simulink model "StateSpaceExeAntiWindup"  (Simulink 7.8)
settings: Solver=ode45  SolverMode=SingleTasking  StartTime=0.0  StopTime=50  RelTol=1e-3
values from neighbouring files (symbols this model uses):
  A = [-7.6258  0; 1  0]    [stateSpaceData.mat]
  B = [1 0]    [stateSpaceData.mat]
  C = [0 162.7435]    [stateSpaceData.mat]
  D = 0    [stateSpaceData.mat]
  K = [-1.6258 11]    [stateSpaceData.mat]    (also in toStateSpace.m = [Kx(1) Kx(2)]; toStateSpaceAntiWindup.m = [Kx(1) Kx(2)])
  Ki = 0.036867831895    [stateSpaceData.mat]    (also in toStateSpace.m = -Kx(3); toStateSpaceAntiWindup.m = -Kx(3))
  L = [80.8124614847 1.48930187688]    [stateSpaceData.mat]    (also in toStateSpace.m = acker(A', C', [polo1, polo2])'; toStateSpaceAntiWindup.m = acker(A', C', [polo1, polo2])')
settings Model: Creator=lucas  LastModifiedBy=lucas  CovMetricSettings=dwe  CovHtmlReporting=off  covSaveCumulativeToWorkspaceVar=off  CovSaveSingleToWorkspaceVar=off  CovExternalEMLEnable=on
settings DataIOCC: LimitDataPoints=off  SaveFormat=StructureWithTime  SignalLoggingSaveFormat=Dataset
settings OptimizationCC: ExpressionDepthLimit=128
settings DebuggingCC: UnderspecifiedInitializationDetection=Simplified  MergeDetectMultiDrivingBlocksExec=error  SolverPrmCheckMsg=none  FrameProcessingCompatibilityMsg=error  StateNameClashWarn=none  SFUnexpectedBacktrackingDiag=error  SFNoUnconditionalDefaultTransitionDiag=error
settings HardwareCC: ProdBitPerPointer=64  ProdLargestAtomicFloat=Float  ProdIntDivRoundTo=Zero  ProdEndianess=LittleEndian  ProdHWDeviceType=Specified
settings SFSimCC: SimUseLocalCustomCode=on
settings RTWCC: RTWUseLocalCustomCode=on
settings CodeAppCC: CustomSymbolStrType=$N$R$M_T
settings GRTTargetCC: TargetFunctionLibrary=C99 (ISO)  GeneratePreprocessorConditionals=Use local settings

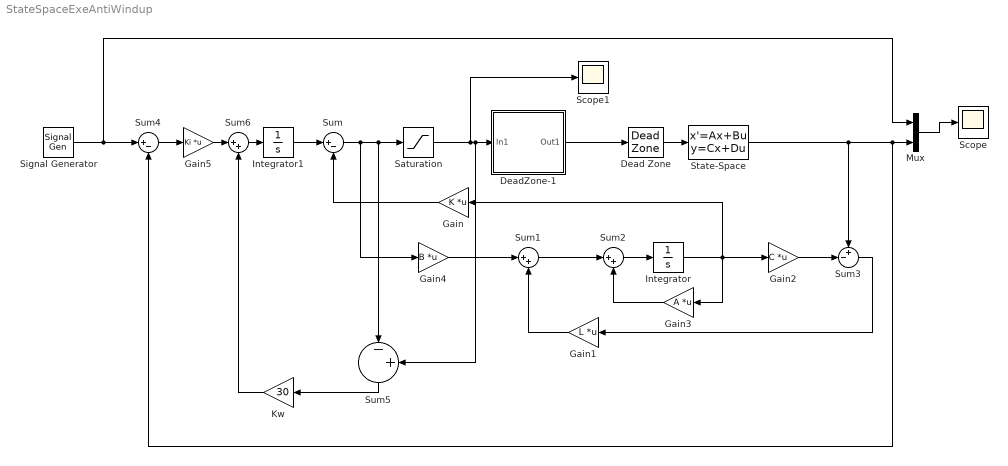
== system StateSpaceExeAntiWindup ==
  Dead Zone : DeadZone  LowerValue=-0.02695  UpperValue=0.5449  ZeroCross=off  SaturateOnIntegerOverflow=on
  DeadZone-1 : Subsystem
  Gain : Gain  Gain=K  Multiplication=Matrix(K*u)
  Gain1 : Gain  Gain=L  Multiplication=Matrix(K*u)
  Gain2 : Gain  Gain=C  Multiplication=Matrix(K*u)
  Gain3 : Gain  Gain=A  Multiplication=Matrix(K*u)
  Gain4 : Gain  Gain=B  Multiplication=Matrix(K*u)
  Gain5 : Gain  Gain=Ki  Multiplication=Matrix(K*u)
  Integrator : Integrator
  Integrator1 : Integrator
  Kw : Gain  Gain=30
  Mux : Mux  Inputs=2
  Saturation : Saturate  UpperLimit=6  LowerLimit=-6
  Scope : Scope
      settings: TimeRange=auto  MaxDataPoints=5000  SaveToWorkspace=off  SaveName=ScopeData  YMin=-201.82571  YMax=211.09069  SampleTime=-1
  Scope1 : Scope
      settings: TimeRange=auto  MaxDataPoints=5000  SaveToWorkspace=off  YMin=-28.32671  YMax=32.53698  SampleTime=-1
  Signal Generator : SignalGenerator  WaveForm=square  Amplitude=200  Frequency=0.1  Units=rad/sec
  State-Space : StateSpace  A=A  B=B  C=C  D=D  X0=0
  Sum : Sum  Inputs=|+-
  Sum1 : Sum  Inputs=|++
  Sum2 : Sum  Inputs=|++
  Sum3 : Sum  Inputs=+-|
  Sum4 : Sum  Inputs=|+-
  Sum5 : Sum  Inputs=|-+
  Sum6 : Sum  Inputs=|++
  wires:
  Mux/1 -> Scope/1
  Sum4/1 -> Gain5/1
  Sum/1 -> Sum5/1, Saturation/1, Gain4/1
  Gain2/1 -> Sum3/2
  Gain3/1 -> Sum2/2
  Sum2/1 -> Integrator/1
  Sum3/1 -> Gain1/1
  Gain1/1 -> Sum1/2
  Sum1/1 -> Sum2/1
  Gain4/1 -> Sum1/1
  Integrator/1 -> Gain/1, Gain3/1, Gain2/1
  Gain/1 -> Sum/2
  Signal Generator/1 -> Mux/1, Sum4/1
  Integrator1/1 -> Sum/1
  Saturation/1 -> Scope1/1, Sum5/2, DeadZone-1/1(In1)
  State-Space/1 -> Sum3/1, Sum4/2, Mux/2
  DeadZone-1/1(Out1) -> Dead Zone/1
  Dead Zone/1 -> State-Space/1
  Gain5/1 -> Sum6/1
  Sum6/1 -> Integrator1/1
  Kw/1 -> Sum6/2
  Sum5/1 -> Kw/1

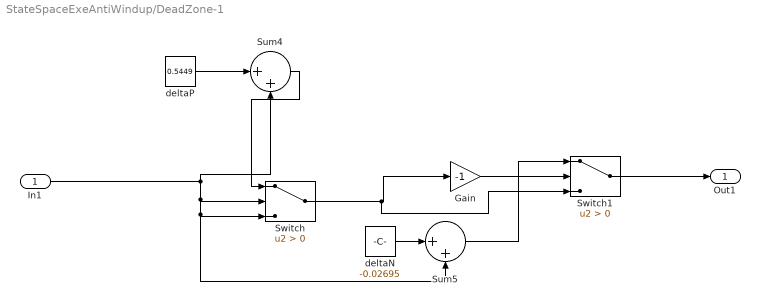
== system StateSpaceExeAntiWindup/DeadZone-1 ==
  In1 : Inport
  Gain : Gain  Gain=-1
  Sum4 : Sum  Inputs=|++
  Sum5 : Sum  Inputs=|++
  Switch : Switch  Criteria=u2 > Threshold
  Switch1 : Switch  Criteria=u2 > Threshold
  deltaN : Constant  Value=-0.02695
  deltaP : Constant  Value=0.5449
  Out1 : Outport
  wires:
  Sum4/1 -> Switch/1
  Switch/1 -> Switch1/3, Gain/1
  Sum5/1 -> Switch1/1
  Gain/1 -> Switch1/2
  deltaN/1 -> Sum5/1
  In1/1 -> Sum4/2, Switch/3, Sum5/2, Switch/2
  Switch1/1 -> Out1/1
  deltaP/1 -> Sum4/1
